simulink library "lib_vehicle"  (Simulink 4.1.1)
undefined symbols (not defined in the file or in its folder): cyc_mph, lib_help, NOTES, veh_air_density, veh_CD, veh_FA, veh_front_wt_frac, veh_gravity, veh_mass, veh_roadwheel_radius, veh_rr_a, veh_rr_alpha, veh_rr_b, veh_rr_beta, veh_rr_c, wh_1st_rrc, wh_2nd_rrc, wh_pressure, wh_radius
libraries: lib_vehicle x23
settings Model: LastModifiedBy=ssprik
settings Model: ModifiedComment=|
  | ssprik -- Fri Sep 05 12:04:31 2003 -- Version 1.64
  | added climbing grade calculation in .../vehicle speed (m/s)/ j2452/c
settings Model: ModifiedHistory=|
  | ssprik -- Fri Sep 05 12:04:31 2003 -- Version 1.64
  | added climbing grade calculation in .../vehicle speed (m/s)/ j2452/c
  | 
  | abrooker -- Fri Feb 07 11:31:15 2003 -- Version 1.63
  | 
  | 
  | abrooker -- Fri Feb 07 11:30:31 2003 -- Version 1.62
  | 
  | 
  | abrooker -- Fri Feb 07 07:46:30 2003 -- Version 1.61
  | 
  | 
  | abrooker -- Thu Feb 06 15:38:07 2003 -- Version 1.60
  | 
  | 
  | abrooker -- Thu Feb 06 14:26:47 2003 -- Version 1.59
  | changed from outputting force to power
  | 
  | abrooker -- Thu Feb 06 13:48:22 2003 -- Version 1.58
  | 
  | 
  | abrooker -- Thu Feb 06 13:42:04 2003 -- Version 1.57
  | 
  | 
  | abrooker -- Wed Feb 05 11:42:46 2003 -- Version 1.56
  | 
  | 
  | abrooker -- Wed Feb 05 11:29:37 2003 -- Version 1.55
  | 
  | 
  | abrooker -- Wed Feb 05 11:27:23 2003 -- Version 1.54
  | 
  | 
  | abrooker -- Wed Feb 05 11:19:28 2003 -- Version 1.53
  | Changed Fr_out to Fr in new rolling resistance block
  | 
  | abrooker -- Wed Feb 05 10:01:32 2003 -- Version 1.52
  | added outputs for Altia
  | 
  | mokeefe -- Thu Apr 18 08:39:48 2002 -- Version 1.51
  | saving the model:
  | o "without the model browser open"
  | o with only top-level screen visible
  | o with "fit to view" enabled
  | o with "status bar" off and "toolbar" off
  | o with "prompt to update model history with each save" on

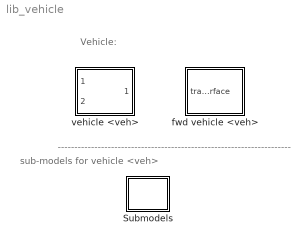
== system lib_vehicle ==
  note: Vehicle:
  note: ----------------------------------------------------------------------
  note: sub-models
      | for vehicle
      | <veh>
  Submodels : Subsystem
      settings: RTWFcnNameOpts=Auto  RTWFileNameOpts=Auto
  fwd vehicle <veh> : Subsystem
      settings: RTWFcnNameOpts=Auto  RTWFileNameOpts=Auto
      mask Display: image(imread('bdi_veh.jpg'))
  vehicle <veh> : Subsystem
      settings: RTWFcnNameOpts=Auto  RTWFileNameOpts=Auto
      mask Display: image(imread('bdi_veh.jpg'))

== system lib_vehicle/Submodels ==
  current veh mass : Subsystem
      settings: RTWFcnNameOpts=Auto  RTWFileNameOpts=Auto
  force req'd to overcome rolling resistance (N) : Subsystem
      settings: RTWFcnNameOpts=Auto  RTWFileNameOpts=Auto
  force req'd to overcome rolling resistance (N) j2452 : Subsystem
      settings: RTWFcnNameOpts=Auto  RTWFileNameOpts=Auto
  rolling resistance force : Subsystem  BlockChoice=force req'd to overcome rolling resistance (N)
      settings: TemplateBlock=self  MemberBlocks=force req'd to overcome rolling resistance (N),force req'd to overcome rolling resistance (N) j2452  RTWFcnNameOpts=Auto  RTWFileNameOpts=Auto
  vehicle speed : Subsystem  BlockChoice=vehicle speed (m/s)
      settings: TemplateBlock=self  MemberBlocks=vehicle speed (m/s),vehicle speed (m/s) j2452  RTWFcnNameOpts=Auto  RTWFileNameOpts=Auto
  vehicle speed (m/s) : Subsystem
      settings: RTWFcnNameOpts=Auto  RTWFileNameOpts=Auto
  vehicle speed (m/s) j2452 : Subsystem  AncestorBlock=|
      | lib_vehicle/Submodels/vehicle speed
      |  (m//s) j2452
      settings: RTWFcnNameOpts=Auto  RTWFileNameOpts=Auto

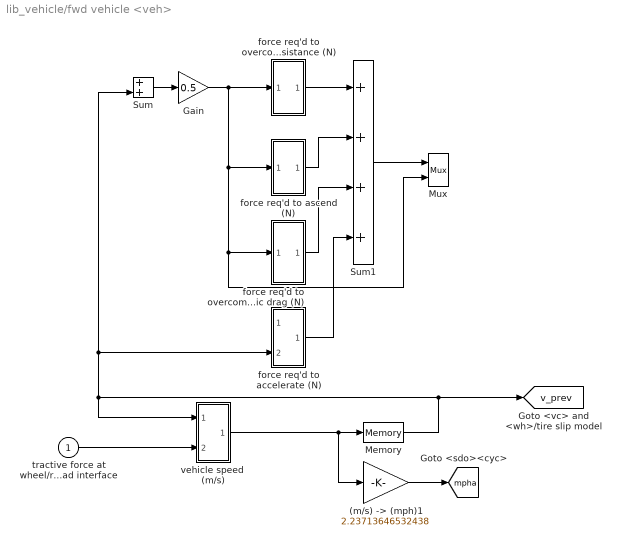
== system lib_vehicle/fwd vehicle <veh> ==
  tractive force at wheel/road interface : Inport  Port=1  LatchInput=off
  "(m/s) -> (mph)1" : Gain  Gain=2.23713646532438  Multiplication=Element-wise(K.*u)  SaturateOnIntegerOverflow=on
  Gain : Gain  Gain=0.5  Multiplication=Element-wise(K.*u)  SaturateOnIntegerOverflow=on
  Memory : Memory  X0=cyc_mph(1,2)*.447  InheritSampleTime=off
      settings: RTWStateStorageClass=Auto
  Mux : Mux  Inputs=2
      settings: DisplayOption=none
  Sum : Sum  Inputs=++  SaturateOnIntegerOverflow=on
  Sum1 : Sum  Inputs=++++  SaturateOnIntegerOverflow=on
  force req'd to accelerate (N) : Subsystem
      settings: RTWFcnNameOpts=Auto  RTWFileNameOpts=Auto
  force req'd to ascend (N) : Subsystem
      settings: RTWFcnNameOpts=Auto  RTWFileNameOpts=Auto
  force req'd to overcome aerodynamic drag (N) : Subsystem
      settings: RTWFcnNameOpts=Auto  RTWFileNameOpts=Auto
  force req'd to overcome rolling resistance (N) : Subsystem
      settings: RTWFcnNameOpts=Auto  RTWFileNameOpts=Auto
  vehicle speed  (m/s) : Subsystem
      settings: RTWFcnNameOpts=Auto  RTWFileNameOpts=Auto
  tag scope: mpha=global, v_prev=global
  wires:
  vehicle speed  (m/s)/1(vehicle speed achieved at end of time step (m/s)) -> Memory/1, "(m/s) -> (mph)1"/1
  Gain/1 -> force req'd to overcome rolling resistance (N)/1(average vehicle speed over time step (m/s)), force req'd to overcome aerodynamic drag (N)/1(average vehicle speed over time step (m/s)), Mux/2, force req'd to ascend (N)/1(average vehicle speed over time step (m/s))
  Sum/1 -> Gain/1
  force req'd to overcome aerodynamic drag (N)/1(D aero(N)) -> Sum1/3
  force req'd to accelerate (N)/1((N)) -> Sum1/4
  Memory/1 -> force req'd to accelerate (N)/2(v prev), Sum/2, vehicle speed  (m/s)/1(vehicle speed at beginning of time step (m/s)), [v_prev]
  "(m/s) -> (mph)1"/1 -> [mpha]
  force req'd to ascend (N)/1((N)) -> Sum1/2
  force req'd to overcome rolling resistance (N)/1((N)) -> Sum1/1
  tractive force at wheel/road interface/1 -> vehicle speed  (m/s)/2(available tractive force (N))
  Sum1/1 -> Mux/1

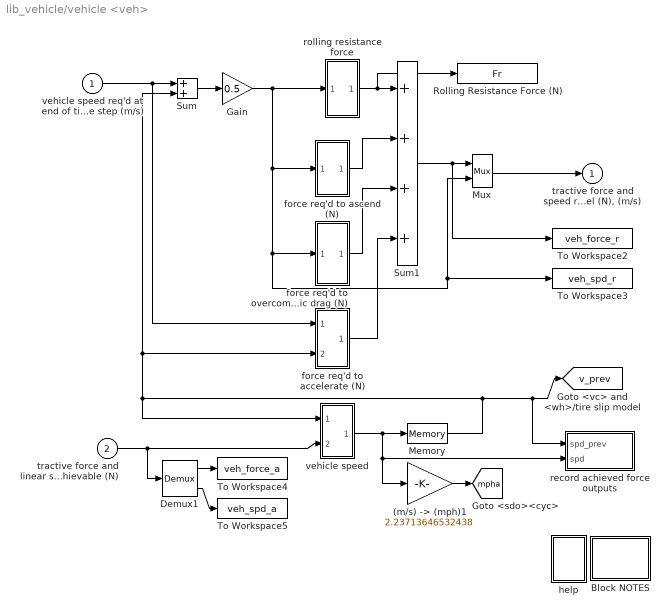
== system lib_vehicle/vehicle <veh> ==
  vehicle speed req'd at end of time step (m/s) : Inport  Port=1  LatchInput=off
  tractive force and linear speed achievable (N) : Inport  Port=2  LatchInput=off
  "(m/s) -> (mph)1" : Gain  Gain=2.23713646532438  Multiplication=Element-wise(K.*u)  SaturateOnIntegerOverflow=on
  Block NOTES : Subsystem
      settings: RTWFcnNameOpts=Auto  RTWFileNameOpts=Auto
      mask Display: disp('Block\nNOTES')
  Demux1 : Demux  Outputs=2  BusSelectionMode=off
  Gain : Gain  Gain=0.5  Multiplication=Element-wise(K.*u)  SaturateOnIntegerOverflow=on
  Memory : Memory  X0=cyc_mph(1,2)*.447  InheritSampleTime=off
      settings: RTWStateStorageClass=Auto
  Mux : Mux  Inputs=2
      settings: DisplayOption=none
  Rolling Resistance Force (N) : ToWorkspace  VariableName=Fr  SampleTime=-1  SaveFormat=Array
  Sum : Sum  Inputs=++  SaturateOnIntegerOverflow=on
  Sum1 : Sum  Inputs=++++  SaturateOnIntegerOverflow=on
  To Workspace2 : ToWorkspace  VariableName=veh_force_r  SampleTime=-1  SaveFormat=Array
  To Workspace3 : ToWorkspace  VariableName=veh_spd_r  SampleTime=-1  SaveFormat=Array
  To Workspace4 : ToWorkspace  VariableName=veh_force_a  SampleTime=-1  SaveFormat=Array
  To Workspace5 : ToWorkspace  VariableName=veh_spd_a  SampleTime=-1  SaveFormat=Array
  force req'd to accelerate (N) : Subsystem
      settings: RTWFcnNameOpts=Auto  RTWFileNameOpts=Auto
  force req'd to ascend (N) : Subsystem
      settings: RTWFcnNameOpts=Auto  RTWFileNameOpts=Auto
  force req'd to overcome aerodynamic drag (N) : Subsystem
      settings: RTWFcnNameOpts=Auto  RTWFileNameOpts=Auto
  help : Subsystem
      settings: OpenFcn=web(['file:\\\' which('vehicle.htm')]);  RTWFcnNameOpts=Auto  RTWFileNameOpts=Auto
      mask Display: image(imread('doc_man.jpg'))
  record achieved force outputs : Subsystem
      settings: RTWFcnNameOpts=Auto  RTWFileNameOpts=Auto
  rolling resistance force : Subsystem  BlockChoice=force req'd to overcome rolling resistance (N)
      settings: AttributesFormatString=%<BlockChoice>  TemplateBlock=lib_vehicle/Submodels/rolling resistance force  MemberBlocks=force req'd to overcome rolling resistance (N),force req'd to overcome rolling resistance (N) j2452  RTWFcnNameOpts=Auto  RTWFileNameOpts=Auto
  vehicle speed : Subsystem  BlockChoice=vehicle speed (m/s)
      settings: AttributesFormatString=%<BlockChoice>  TemplateBlock=lib_vehicle/Submodels/vehicle speed  MemberBlocks=vehicle speed (m/s),vehicle speed (m/s) j2452  RTWFcnNameOpts=Auto  RTWFileNameOpts=Auto
  "tractive force and speed required of tire and wheel (N), (m/s)" : Outport  Port=1  InitialOutput=0
  tag scope: mpha=global, v_prev=global
  wires:
  rolling resistance force/1(Fr (N)) -> Sum1/1, Rolling Resistance Force (N)/1
  force req'd to ascend (N)/1((N)) -> Sum1/2
  "(m/s) -> (mph)1"/1 -> [mpha]
  Memory/1 -> Sum/2, force req'd to accelerate (N)/2(v prev), vehicle speed/1(vehicle speed at beginning of time step (m/s)), [v_prev], record achieved force outputs/1(spd_prev)
  force req'd to accelerate (N)/1((N)) -> Sum1/4
  force req'd to overcome aerodynamic drag (N)/1(D aero(N)) -> Sum1/3
  Demux1/2 -> To Workspace5/1
  Demux1/1 -> To Workspace4/1
  Sum1/1 -> To Workspace2/1, Mux/1
  Mux/1 -> "tractive force and speed required of tire and wheel (N), (m/s)"/1
  vehicle speed req'd at end of time step (m/s)/1 -> Sum/1, force req'd to accelerate (N)/1(v(m/s))
  Sum/1 -> Gain/1
  Gain/1 -> force req'd to ascend (N)/1(average vehicle speed over time step (m/s)), To Workspace3/1, Mux/2, force req'd to overcome aerodynamic drag (N)/1(average vehicle speed over time step (m/s)), rolling resistance force/1(average vehicle speed over time step (m/s))
  tractive force and linear speed achievable (N)/1 -> Demux1/1, vehicle speed/2("available tractive force and linear speed (N), (m/s)")
  vehicle speed/1(vehicle speed achievable at end of time step (m/s)) -> Memory/1, "(m/s) -> (mph)1"/1, record achieved force outputs/2(spd)

== system lib_vehicle/Submodels/current veh mass ==
  Constant3 : Constant  Value=veh_mass
  Sum1 : Sum  Inputs=|++  SaturateOnIntegerOverflow=on
  Out1 : Outport  Port=1
  wires:
  Sum1/1 -> Out1/1
  [veh_cargo_mass] -> Sum1/2
  Constant3/1 -> Sum1/1

== system lib_vehicle/Submodels/force req'd to overcome rolling resistance (N) ==
  average vehicle speed over time step (m/s) : Inport  Port=1  LatchInput=off
  Constant : Constant  Value=wh_1st_rrc
  Constant1 : Constant  Orientation=up  Value=0
  Constant2 : Constant  Orientation=left  Value=veh_gravity
  Gain1 : Gain  Gain=wh_2nd_rrc  Multiplication=Element-wise(K.*u)  SaturateOnIntegerOverflow=on
  Product : Product  Inputs=4  Multiplication=Element-wise(.*)  SaturateOnIntegerOverflow=on
  Sum : Sum  Inputs=++  SaturateOnIntegerOverflow=on
  Switch : Switch  Threshold=eps
  Trig Fn2 : Trigonometry  Operator=atan  OutputSignalType=auto
  Trig Fn3 : Trigonometry  Operator=cos  OutputSignalType=auto
  current veh mass : lib_vehicle/Submodels/current veh mass
      settings: RTWFcnNameOpts=Auto  RTWFileNameOpts=Auto
  Fr (N) : Outport  Port=1  InitialOutput=0
  wires:
  Trig Fn2/1 -> Trig Fn3/1
  [grade] -> Trig Fn2/1
  current veh mass/1 -> Product/4
  Trig Fn3/1 -> Product/3
  Product/1 -> Switch/1
  Constant2/1 -> Product/1
  Sum/1 -> Product/2
  Constant1/1 -> Switch/3
  average vehicle speed over time step (m/s)/1 -> Switch/2, Gain1/1
  Switch/1 -> Fr (N)/1
  Gain1/1 -> Sum/2
  Constant/1 -> Sum/1

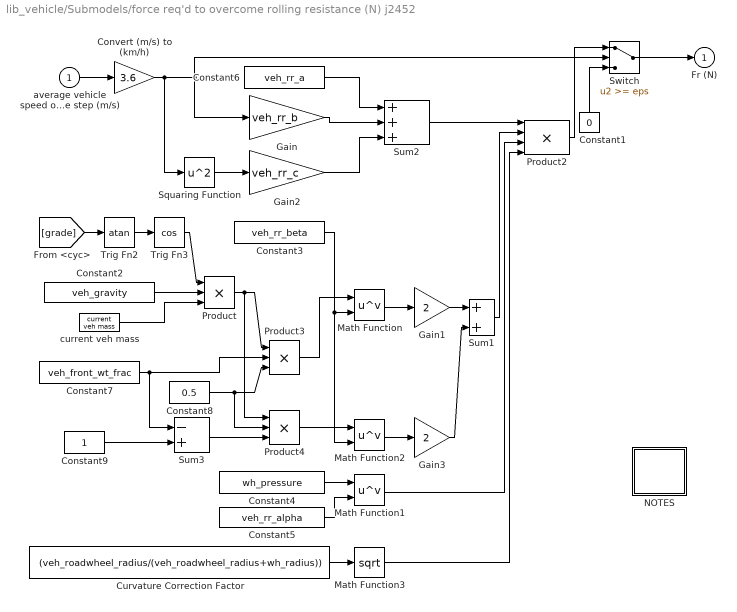
== system lib_vehicle/Submodels/force req'd to overcome rolling resistance (N) j2452 ==
  average vehicle speed over time step (m/s) : Inport  Port=1  LatchInput=off
  Constant1 : Constant  Orientation=up  Value=0
  Constant2 : Constant  Value=veh_gravity
  Constant3 : Constant  Value=veh_rr_beta
  Constant4 : Constant  Value=wh_pressure
  Constant5 : Constant  Value=veh_rr_alpha
  Constant6 : Constant  Value=veh_rr_a
  Constant7 : Constant  Value=veh_front_wt_frac
  Constant8 : Constant  Value=0.5
  Constant9 : Constant  Value=1
  Convert (m/s) to (km/h) : Gain  Description=Conversion of m/s to km/h  Gain=3.6  Multiplication=Element-wise(K.*u)  SaturateOnIntegerOverflow=on
  Curvature Correction Factor : Constant  Value=(veh_roadwheel_radius/(veh_roadwheel_radius+wh_radius))
  Gain : Gain  Gain=veh_rr_b  Multiplication=Element-wise(K.*u)  SaturateOnIntegerOverflow=on
  Gain1 : Gain  Gain=2  Multiplication=Element-wise(K.*u)  SaturateOnIntegerOverflow=on
  Gain2 : Gain  Gain=veh_rr_c  Multiplication=Element-wise(K.*u)  SaturateOnIntegerOverflow=on
  Gain3 : Gain  Gain=2  Multiplication=Element-wise(K.*u)  SaturateOnIntegerOverflow=on
  Math Function : Math  Operator=pow  OutputSignalType=auto
  Math Function1 : Math  Operator=pow  OutputSignalType=auto
  Math Function2 : Math  Operator=pow  OutputSignalType=auto
  Math Function3 : Math  Operator=sqrt  OutputSignalType=auto
  NOTES : Subsystem  Description=Notes  Orientation=left  AncestorBlock=lib_help/NOTES
      settings: RTWFcnNameOpts=Auto  RTWFileNameOpts=Auto
      mask Display: disp('Block\nNOTES')
  Product : Product  Inputs=3  Multiplication=Element-wise(.*)  SaturateOnIntegerOverflow=on
  Product2 : Product  Inputs=4  Multiplication=Element-wise(.*)  SaturateOnIntegerOverflow=on
  Product3 : Product  Inputs=3  Multiplication=Element-wise(.*)  SaturateOnIntegerOverflow=on
  Product4 : Product  Inputs=3  Multiplication=Element-wise(.*)  SaturateOnIntegerOverflow=on
  Squaring Function : Math  Operator=square  OutputSignalType=auto
  Sum1 : Sum  Inputs=++  SaturateOnIntegerOverflow=on
  Sum2 : Sum  Inputs=+++  SaturateOnIntegerOverflow=on
  Sum3 : Sum  Inputs=-+  SaturateOnIntegerOverflow=on
  Switch : Switch  Threshold=eps
  Trig Fn2 : Trigonometry  Operator=atan  OutputSignalType=auto
  Trig Fn3 : Trigonometry  Operator=cos  OutputSignalType=auto
  current veh mass : lib_vehicle/Submodels/current veh mass
      settings: RTWFcnNameOpts=Auto  RTWFileNameOpts=Auto
  Fr (N) : Outport  Port=1  InitialOutput=0
  wires:
  Curvature Correction Factor/1 -> Math Function3/1
  Math Function3/1 -> Product2/4
  Constant3/1 -> Math Function2/2, Math Function/2
  Convert (m/s) to (km/h)/1 -> Switch/2, Gain/1, Squaring Function/1
  average vehicle speed over time step (m/s)/1 -> Convert (m/s) to (km/h)/1
  Constant5/1 -> Math Function1/2
  Sum2/1 -> Product2/1
  Sum1/1 -> Product2/2
  Math Function1/1 -> Product2/3
  Gain3/1 -> Sum1/2
  Math Function2/1 -> Gain3/1
  Product4/1 -> Math Function2/1
  Sum3/1 -> Product4/3
  Constant9/1 -> Sum3/2
  Gain1/1 -> Sum1/1
  Product3/1 -> Math Function/1
  Constant8/1 -> Product4/2, Product3/3
  Constant7/1 -> Sum3/1, Product3/2
  Product/1 -> Product4/1, Product3/1
  Switch/1 -> Fr (N)/1
  Product2/1 -> Switch/1
  Gain2/1 -> Sum2/3
  Gain/1 -> Sum2/2
  Constant6/1 -> Sum2/1
  Squaring Function/1 -> Gain2/1
  Math Function/1 -> Gain1/1
  Constant4/1 -> Math Function1/1
  current veh mass/1 -> Product/3
  Constant2/1 -> Product/2
  Trig Fn3/1 -> Product/1
  [grade] -> Trig Fn2/1
  Constant1/1 -> Switch/3
  Trig Fn2/1 -> Trig Fn3/1

== system lib_vehicle/Submodels/rolling resistance force ==
  average vehicle speed over time step (m/s) : Inport  Port=1  LatchInput=off
  force req'd to overcome rolling resistance (N) : lib_vehicle/Submodels/force req'd to overcome rolling resistance (N)
      settings: RTWFcnNameOpts=Auto  RTWFileNameOpts=Auto
  Fr (N) : Outport  Port=1
  wires:
  average vehicle speed over time step (m/s)/1 -> force req'd to overcome rolling resistance (N)/1
  force req'd to overcome rolling resistance (N)/1 -> Fr (N)/1

== system lib_vehicle/Submodels/vehicle speed ==
  vehicle speed at beginning of time step (m/s) : Inport  Port=1  LatchInput=off
  "available tractive force and linear speed (N), (m/s)" : Inport  Port=2  LatchInput=off
  vehicle speed (m/s) : lib_vehicle/Submodels/vehicle speed (m//s)
      settings: RTWFcnNameOpts=Auto  RTWFileNameOpts=Auto
  vehicle speed achievable at end of time step (m/s) : Outport  Port=1
  wires:
  vehicle speed at beginning of time step (m/s)/1 -> vehicle speed (m/s)/1
  "available tractive force and linear speed (N), (m/s)"/1 -> vehicle speed (m/s)/2
  vehicle speed (m/s)/1 -> vehicle speed achievable at end of time step (m/s)/1

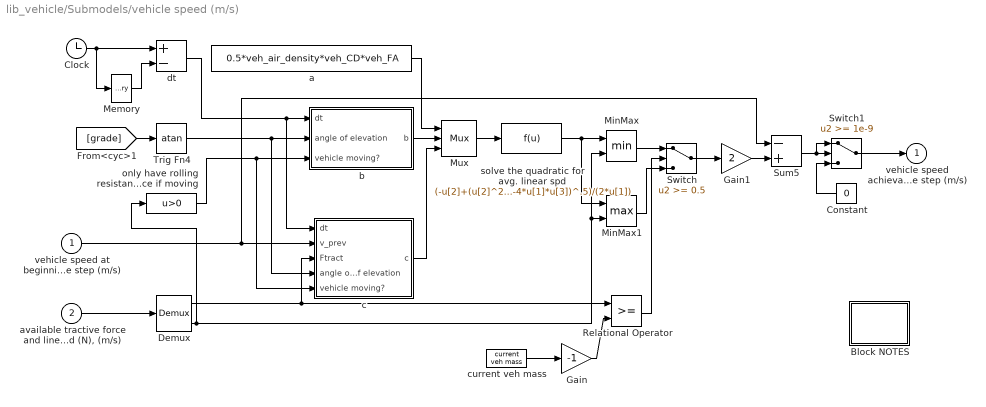
== system lib_vehicle/Submodels/vehicle speed (m/s) ==
  vehicle speed at beginning of time step (m/s) : Inport  Port=1  LatchInput=off
  "available tractive force and linear speed (N), (m/s)" : Inport  Port=2  LatchInput=off
  Block NOTES : Subsystem
      settings: RTWFcnNameOpts=Auto  RTWFileNameOpts=Auto
      mask Display: disp('Block\nNOTES')
  Clock : Clock
      settings: DisplayTime=off  Decimation=10
  Constant : Constant  Orientation=left  Value=0
  Demux : Demux  Outputs=2  BusSelectionMode=off
  Gain : Gain  Gain=-1  Multiplication=Element-wise(K.*u)  SaturateOnIntegerOverflow=on
  Gain1 : Gain  Gain=2  Multiplication=Element-wise(K.*u)  SaturateOnIntegerOverflow=on
  Memory : Memory  X0=-.1  InheritSampleTime=off
      settings: RTWStateStorageClass=Auto
  MinMax : MinMax  Function=min  Inputs=2
  MinMax1 : MinMax  Function=max  Inputs=2
  Mux : Mux  Inputs=3
      settings: DisplayOption=none
  Relational Operator : RelationalOperator  Operator=>=
  Sum5 : Sum  Inputs=-+  SaturateOnIntegerOverflow=on
  Switch : Switch  Threshold=0.5
  Switch1 : Switch  Threshold=1e-9
  Trig Fn4 : Trigonometry  Operator=atan  OutputSignalType=auto
  a : Constant  Value=0.5*veh_air_density*veh_CD*veh_FA
  b : Subsystem
      settings: RTWFcnNameOpts=Auto  RTWFileNameOpts=Auto
  c : Subsystem
      settings: RTWFcnNameOpts=Auto  RTWFileNameOpts=Auto
  current veh mass : lib_vehicle/Submodels/current veh mass
      settings: RTWFcnNameOpts=Auto  RTWFileNameOpts=Auto
  dt : Sum  Inputs=+-  SaturateOnIntegerOverflow=on
  only have rolling resistance if moving : Fcn  Expr=u>0
  solve the quadratic for avg. linear spd : Fcn  Expr=(-u[2]+(u[2]^2-4*u[1]*u[3])^.5)/(2*u[1])
  vehicle speed achievable at end of time step (m/s) : Outport  Port=1  InitialOutput=0
  wires:
  Relational Operator/1 -> Switch/2
  current veh mass/1 -> Gain/1
  Gain/1 -> Relational Operator/2
  Switch/1 -> Gain1/1
  solve the quadratic for avg. linear spd/1 -> MinMax/1, MinMax1/1
  Gain1/1 -> Sum5/2
  MinMax1/1 -> Switch/3
  MinMax/1 -> Switch/1
  a/1 -> Mux/1
  Mux/1 -> solve the quadratic for avg. linear spd/1
  Switch1/1 -> vehicle speed achievable at end of time step (m/s)/1
  b/1(b) -> Mux/2
  Clock/1 -> dt/1, Memory/1
  Memory/1 -> dt/2
  [grade] -> Trig Fn4/1
  dt/1 -> b/1(dt), c/1(dt)
  Trig Fn4/1 -> b/2(angle of elevation), c/4(angle of elevation)
  only have rolling resistance if moving/1 -> b/3(vehicle moving?), c/5(vehicle moving?)
  Sum5/1 -> Switch1/1, Switch1/2
  Constant/1 -> Switch1/3
  "available tractive force and linear speed (N), (m/s)"/1 -> Demux/1
  c/1(c) -> Mux/3
  Demux/2 -> only have rolling resistance if moving/1, MinMax/2, MinMax1/2
  Demux/1 -> Relational Operator/1, c/3(Ftract)
  vehicle speed at beginning of time step (m/s)/1 -> c/2(v_prev), Sum5/1

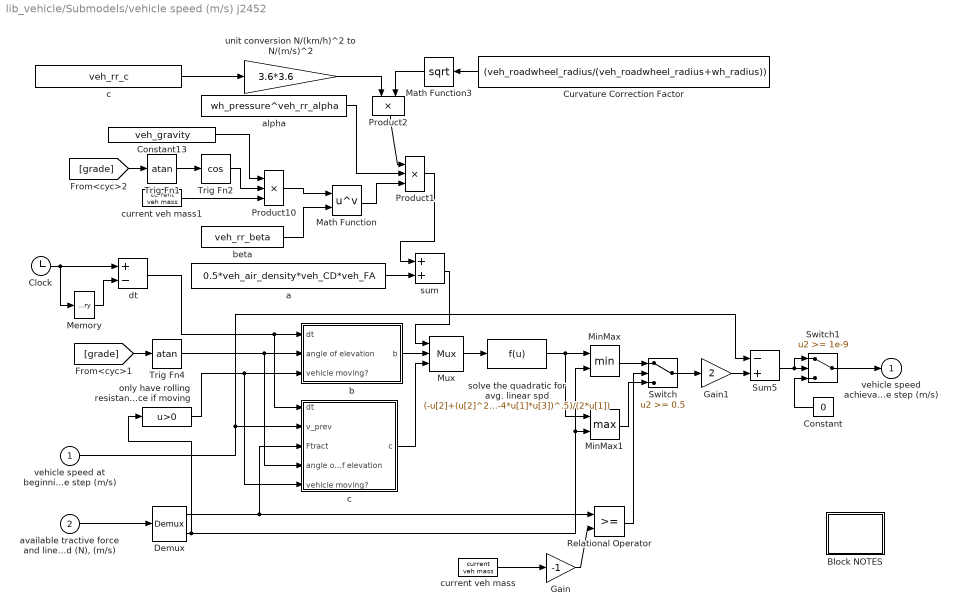
== system lib_vehicle/Submodels/vehicle speed (m/s) j2452 ==
  vehicle speed at beginning of time step (m/s) : Inport  Port=1  LatchInput=off
  "available tractive force and linear speed (N), (m/s)" : Inport  Port=2  LatchInput=off
  Block NOTES : Subsystem
      settings: RTWFcnNameOpts=Auto  RTWFileNameOpts=Auto
      mask Display: disp('Block\nNOTES')
  Clock : Clock
      settings: DisplayTime=off  Decimation=10
  Constant : Constant  Orientation=left  Value=0
  Constant13 : Constant  Value=veh_gravity
  Curvature Correction Factor : Constant  Orientation=left  Value=(veh_roadwheel_radius/(veh_roadwheel_radius+wh_radius))  VectorParams1D=off
  Demux : Demux  Outputs=2  BusSelectionMode=off
  Gain : Gain  Gain=-1  Multiplication=Element-wise(K.*u)  SaturateOnIntegerOverflow=on
  Gain1 : Gain  Gain=2  Multiplication=Element-wise(K.*u)  SaturateOnIntegerOverflow=on
  Math Function : Math  Operator=pow  OutputSignalType=auto
  Math Function3 : Math  Orientation=left  Operator=sqrt  OutputSignalType=auto
  Memory : Memory  X0=-.1  InheritSampleTime=off
      settings: RTWStateStorageClass=Auto
  MinMax : MinMax  Function=min  Inputs=2
  MinMax1 : MinMax  Function=max  Inputs=2
  Mux : Mux  Inputs=3
      settings: DisplayOption=none
  Product1 : Product  Inputs=3  Multiplication=Element-wise(.*)  SaturateOnIntegerOverflow=on
  Product10 : Product  Inputs=3  Multiplication=Element-wise(.*)  SaturateOnIntegerOverflow=on
  Product2 : Product  Orientation=down  Inputs=2  Multiplication=Element-wise(.*)  SaturateOnIntegerOverflow=on
  Relational Operator : RelationalOperator  Operator=>=
  Sum5 : Sum  Inputs=-+  SaturateOnIntegerOverflow=on
  Switch : Switch  Threshold=0.5
  Switch1 : Switch  Threshold=1e-9
  Trig Fn1 : Trigonometry  Operator=atan  OutputSignalType=auto
  Trig Fn2 : Trigonometry  Operator=cos  OutputSignalType=auto
  Trig Fn4 : Trigonometry  Operator=atan  OutputSignalType=auto
  a : Constant  Value=0.5*veh_air_density*veh_CD*veh_FA
  alpha : Constant  Value=wh_pressure^veh_rr_alpha
  b : Subsystem
      settings: RTWFcnNameOpts=Auto  RTWFileNameOpts=Auto
  beta : Constant  Value=veh_rr_beta
  c : Subsystem
      settings: RTWFcnNameOpts=Auto  RTWFileNameOpts=Auto
  "c " : Constant  Value=veh_rr_c
  current veh mass : lib_vehicle/Submodels/current veh mass
      settings: RTWFcnNameOpts=Auto  RTWFileNameOpts=Auto
  current veh mass1 : lib_vehicle/Submodels/current veh mass
      settings: RTWFcnNameOpts=Auto  RTWFileNameOpts=Auto
  dt : Sum  Inputs=+-  SaturateOnIntegerOverflow=on
  only have rolling resistance if moving : Fcn  Expr=u>0
  solve the quadratic for avg. linear spd : Fcn  Expr=(-u[2]+(u[2]^2-4*u[1]*u[3])^.5)/(2*u[1])
  sum : Sum  Inputs=++  SaturateOnIntegerOverflow=on
  unit conversion N/(km/h)^2 to N/(m/s)^2 : Gain  Gain=3.6*3.6  Multiplication=Element-wise(K.*u)  SaturateOnIntegerOverflow=on
  vehicle speed achievable at end of time step (m/s) : Outport  Port=1  InitialOutput=0
  wires:
  Product2/1 -> Product1/1
  Math Function3/1 -> Product2/2
  unit conversion N/(km/h)^2 to N/(m/s)^2/1 -> Product2/1
  Curvature Correction Factor/1 -> Math Function3/1
  current veh mass1/1 -> Product10/3
  Trig Fn2/1 -> Product10/2
  Constant13/1 -> Product10/1
  Product1/1 -> sum/1
  Math Function/1 -> Product1/3
  alpha/1 -> Product1/2
  "c "/1 -> unit conversion N/(km/h)^2 to N/(m/s)^2/1
  sum/1 -> Mux/1
  a/1 -> sum/2
  beta/1 -> Math Function/2
  Product10/1 -> Math Function/1
  Trig Fn1/1 -> Trig Fn2/1
  [grade] -> Trig Fn1/1
  vehicle speed at beginning of time step (m/s)/1 -> c/2(v_prev), Sum5/1
  Demux/1 -> c/3(Ftract), Relational Operator/1
  Demux/2 -> MinMax1/2, MinMax/2, only have rolling resistance if moving/1
  c/1(c) -> Mux/3
  "available tractive force and linear speed (N), (m/s)"/1 -> Demux/1
  Constant/1 -> Switch1/3
  Sum5/1 -> Switch1/2, Switch1/1
  only have rolling resistance if moving/1 -> c/5(vehicle moving?), b/3(vehicle moving?)
  Trig Fn4/1 -> c/4(angle of elevation), b/2(angle of elevation)
  dt/1 -> c/1(dt), b/1(dt)
  [grade] -> Trig Fn4/1
  Memory/1 -> dt/2
  Clock/1 -> Memory/1, dt/1
  b/1(b) -> Mux/2
  Switch1/1 -> vehicle speed achievable at end of time step (m/s)/1
  Mux/1 -> solve the quadratic for avg. linear spd/1
  MinMax/1 -> Switch/1
  MinMax1/1 -> Switch/3
  Gain1/1 -> Sum5/2
  solve the quadratic for avg. linear spd/1 -> MinMax1/1, MinMax/1
  Switch/1 -> Gain1/1
  Gain/1 -> Relational Operator/2
  current veh mass/1 -> Gain/1
  Relational Operator/1 -> Switch/2

== system lib_vehicle/fwd vehicle <veh>/force req'd to accelerate (N) ==
  v(m/s) : Inport  Port=1  LatchInput=off
  v prev : Inport  Port=2  LatchInput=off
  Clock : Clock
      settings: DisplayTime=off  Decimation=10
  Constant : Constant  Value=veh_mass
  Memory : Memory  X0=-0.1  InheritSampleTime=off
      settings: RTWStateStorageClass=Auto
  Product1 : Product  Inputs=**/  Multiplication=Element-wise(.*)  SaturateOnIntegerOverflow=on
  Sum : Sum  Inputs=+-  SaturateOnIntegerOverflow=on
  Sum1 : Sum  Inputs=+-  SaturateOnIntegerOverflow=on
  (N) : Outport  Port=1  InitialOutput=0
  wires:
  Constant/1 -> Product1/1
  Clock/1 -> Sum1/1, Memory/1
  Memory/1 -> Sum1/2
  Product1/1 -> (N)/1
  v prev/1 -> Sum/2
  v(m/s)/1 -> Sum/1
  Sum1/1 -> Product1/3
  Sum/1 -> Product1/2

== system lib_vehicle/fwd vehicle <veh>/force req'd to ascend (N) ==
  average vehicle speed over time step (m/s) : Inport  Port=1  LatchInput=off
  Constant : Constant  Value=veh_mass*veh_gravity
  Constant1 : Constant  Value=0
  Product : Product  Inputs=2  Multiplication=Element-wise(.*)  SaturateOnIntegerOverflow=on
  Switch : Switch  Threshold=0
  Trigonometric Function : Trigonometry  Operator=atan  OutputSignalType=auto
  Trigonometric Function1 : Trigonometry  Operator=sin  OutputSignalType=auto
  (N) : Outport  Port=1  InitialOutput=0
  wires:
  average vehicle speed over time step (m/s)/1 -> Switch/2
  Constant1/1 -> Switch/3
  Switch/1 -> (N)/1
  Product/1 -> Switch/1
  Constant/1 -> Product/1
  [grade] -> Trigonometric Function/1
  Trigonometric Function1/1 -> Product/2
  Trigonometric Function/1 -> Trigonometric Function1/1

== system lib_vehicle/fwd vehicle <veh>/force req'd to overcome aerodynamic drag (N) ==
  average vehicle speed over time step (m/s) : Inport  Port=1  LatchInput=off
  Constant : Constant  Value=veh_air_density*veh_CD*veh_FA*0.5
  Product : Product  Inputs=3  Multiplication=Element-wise(.*)  SaturateOnIntegerOverflow=on
  D aero(N) : Outport  Port=1  InitialOutput=0
  wires:
  Product/1 -> D aero(N)/1
  Constant/1 -> Product/3
  average vehicle speed over time step (m/s)/1 -> Product/2, Product/1

== system lib_vehicle/fwd vehicle <veh>/force req'd to overcome rolling resistance (N) ==
  average vehicle speed over time step (m/s) : Inport  Port=1  LatchInput=off
  Constant : Constant  Value=wh_1st_rrc
  Constant1 : Constant  Orientation=up  Value=0
  Constant2 : Constant  Orientation=left  Value=veh_mass*veh_gravity
  Gain1 : Gain  Gain=wh_2nd_rrc  Multiplication=Element-wise(K.*u)  SaturateOnIntegerOverflow=on
  Product : Product  Inputs=3  Multiplication=Element-wise(.*)  SaturateOnIntegerOverflow=on
  Sum : Sum  Inputs=++  SaturateOnIntegerOverflow=on
  Switch : Switch  Threshold=eps
  Trig Fn2 : Trigonometry  Operator=atan  OutputSignalType=auto
  Trig Fn3 : Trigonometry  Operator=cos  OutputSignalType=auto
  (N) : Outport  Port=1  InitialOutput=0
  wires:
  Trig Fn3/1 -> Product/3
  Trig Fn2/1 -> Trig Fn3/1
  [grade] -> Trig Fn2/1
  Product/1 -> Switch/1
  Constant2/1 -> Product/1
  Sum/1 -> Product/2
  Constant1/1 -> Switch/3
  average vehicle speed over time step (m/s)/1 -> Switch/2, Gain1/1
  Switch/1 -> (N)/1
  Gain1/1 -> Sum/2
  Constant/1 -> Sum/1

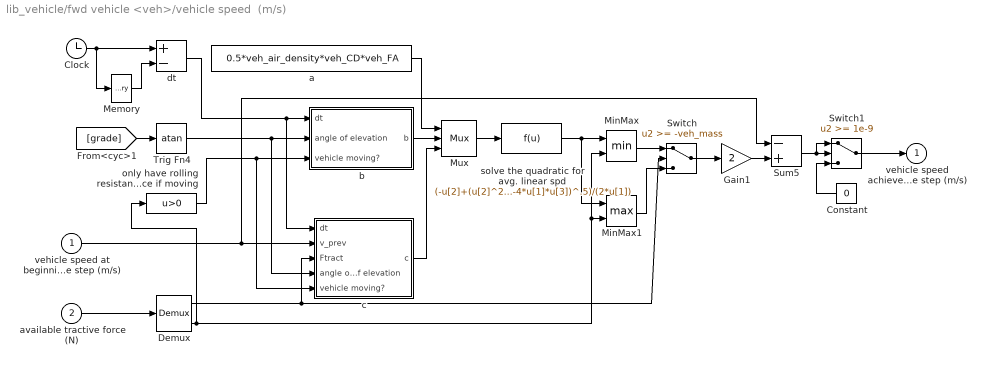
== system lib_vehicle/fwd vehicle <veh>/vehicle speed  (m/s) ==
  vehicle speed at beginning of time step (m/s) : Inport  Port=1  LatchInput=off
  available tractive force (N) : Inport  Port=2  LatchInput=off
  Clock : Clock
      settings: DisplayTime=off  Decimation=10
  Constant : Constant  Orientation=left  Value=0
  Demux : Demux  Outputs=2  BusSelectionMode=off
  Gain1 : Gain  Gain=2  Multiplication=Element-wise(K.*u)  SaturateOnIntegerOverflow=on
  Memory : Memory  X0=-.1  InheritSampleTime=off
      settings: RTWStateStorageClass=Auto
  MinMax : MinMax  Function=min  Inputs=2
  MinMax1 : MinMax  Function=max  Inputs=2
  Mux : Mux  Inputs=3
      settings: DisplayOption=none
  Sum5 : Sum  Inputs=-+  SaturateOnIntegerOverflow=on
  Switch : Switch  Threshold=-veh_mass
  Switch1 : Switch  Threshold=1e-9
  Trig Fn4 : Trigonometry  Operator=atan  OutputSignalType=auto
  a : Constant  Value=0.5*veh_air_density*veh_CD*veh_FA
  b : Subsystem
      settings: RTWFcnNameOpts=Auto  RTWFileNameOpts=Auto
  c : Subsystem
      settings: RTWFcnNameOpts=Auto  RTWFileNameOpts=Auto
  dt : Sum  Inputs=+-  SaturateOnIntegerOverflow=on
  only have rolling resistance if moving : Fcn  Expr=u>0
  solve the quadratic for avg. linear spd : Fcn  Expr=(-u[2]+(u[2]^2-4*u[1]*u[3])^.5)/(2*u[1])
  vehicle speed achieved at end of time step (m/s) : Outport  Port=1  InitialOutput=0
  wires:
  Switch/1 -> Gain1/1
  solve the quadratic for avg. linear spd/1 -> MinMax/1, MinMax1/1
  Gain1/1 -> Sum5/2
  MinMax1/1 -> Switch/3
  MinMax/1 -> Switch/1
  a/1 -> Mux/1
  Mux/1 -> solve the quadratic for avg. linear spd/1
  Switch1/1 -> vehicle speed achieved at end of time step (m/s)/1
  b/1(b) -> Mux/2
  Clock/1 -> dt/1, Memory/1
  Memory/1 -> dt/2
  [grade] -> Trig Fn4/1
  dt/1 -> b/1(dt), c/1(dt)
  Trig Fn4/1 -> b/2(angle of elevation), c/4(angle of elevation)
  only have rolling resistance if moving/1 -> b/3(vehicle moving?), c/5(vehicle moving?)
  Sum5/1 -> Switch1/1, Switch1/2
  Constant/1 -> Switch1/3
  available tractive force (N)/1 -> Demux/1
  c/1(c) -> Mux/3
  Demux/2 -> only have rolling resistance if moving/1, MinMax/2, MinMax1/2
  Demux/1 -> c/3(Ftract), Switch/2
  vehicle speed at beginning of time step (m/s)/1 -> c/2(v_prev), Sum5/1

== system lib_vehicle/vehicle <veh>/Block NOTES ==
  note: Given the tractive force available, this block uses the same equations to determine the achievable speed.
  note: If no drivetrain component ran up against its performance limit during the time step, the achieved speed
      | is taken to be the requested speed.
  note: This block uses the required vehicle speed with vehicle parameters and the previous speed
      | and classic, straightforward equations to determine the tractive force required at the tire/road interface.
  note: A slight simplification, the assumption that (speed_at_end_of_time_step)^2 is roughly equal to
      | (speed_at_end_of_time_step)*(speed_at_beginning_of_time_step), is used to avoid solving
      | a quadratic equation in the solution of v=v(Ftract).

== system lib_vehicle/vehicle <veh>/force req'd to accelerate (N) ==
  v(m/s) : Inport  Port=1  LatchInput=off
  v prev : Inport  Port=2  LatchInput=off
  Clock : Clock
      settings: DisplayTime=off  Decimation=10
  Memory : Memory  X0=-0.1  InheritSampleTime=off
      settings: RTWStateStorageClass=Auto
  Product1 : Product  Inputs=**/  Multiplication=Element-wise(.*)  SaturateOnIntegerOverflow=on
  Sum : Sum  Inputs=+-  SaturateOnIntegerOverflow=on
  Sum1 : Sum  Inputs=+-  SaturateOnIntegerOverflow=on
  current veh mass : lib_vehicle/Submodels/current veh mass
  (N) : Outport  Port=1  InitialOutput=0
  wires:
  Sum/1 -> Product1/2
  Sum1/1 -> Product1/3
  v(m/s)/1 -> Sum/1
  v prev/1 -> Sum/2
  Product1/1 -> (N)/1
  Memory/1 -> Sum1/2
  Clock/1 -> Memory/1, Sum1/1
  current veh mass/1 -> Product1/1

== system lib_vehicle/vehicle <veh>/force req'd to ascend (N) ==
  average vehicle speed over time step (m/s) : Inport  Port=1  LatchInput=off
  Constant : Constant  Value=veh_gravity
  Constant1 : Constant  Value=0
  Product : Product  Inputs=3  Multiplication=Element-wise(.*)  SaturateOnIntegerOverflow=on
  Switch : Switch  Threshold=0
  Trigonometric Function : Trigonometry  Operator=atan  OutputSignalType=auto
  Trigonometric Function1 : Trigonometry  Operator=sin  OutputSignalType=auto
  current veh mass : lib_vehicle/Submodels/current veh mass
      settings: RTWFcnNameOpts=Auto  RTWFileNameOpts=Auto
  (N) : Outport  Port=1  InitialOutput=0
  wires:
  Trigonometric Function/1 -> Trigonometric Function1/1
  Trigonometric Function1/1 -> Product/2
  [grade] -> Trigonometric Function/1
  Constant/1 -> Product/1
  Product/1 -> Switch/1
  Switch/1 -> (N)/1
  Constant1/1 -> Switch/3
  average vehicle speed over time step (m/s)/1 -> Switch/2
  current veh mass/1 -> Product/3

== system lib_vehicle/vehicle <veh>/force req'd to overcome aerodynamic drag (N) ==
  average vehicle speed over time step (m/s) : Inport  Port=1  LatchInput=off
  Constant : Constant  Value=veh_air_density*veh_CD*veh_FA*0.5
  Product : Product  Inputs=3  Multiplication=Element-wise(.*)  SaturateOnIntegerOverflow=on
  D aero(N) : Outport  Port=1  InitialOutput=0
  wires:
  average vehicle speed over time step (m/s)/1 -> Product/1, Product/2
  Constant/1 -> Product/3
  Product/1 -> D aero(N)/1

== system lib_vehicle/vehicle <veh>/help ==

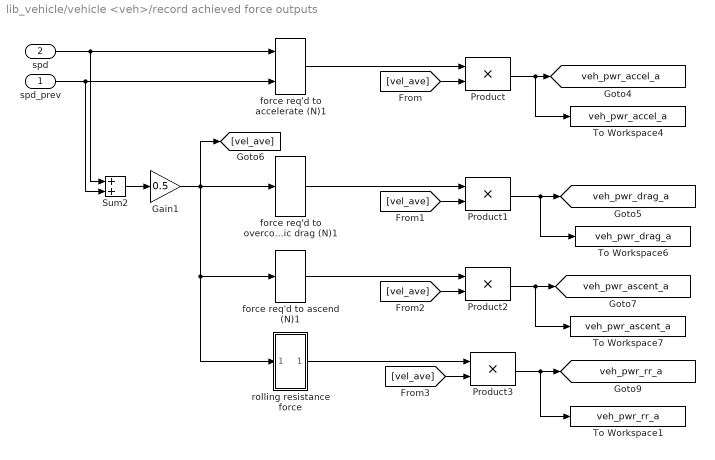
== system lib_vehicle/vehicle <veh>/record achieved force outputs ==
  spd_prev : Inport  Port=1  LatchInput=off
  spd : Inport  Port=2  LatchInput=off
  Gain1 : Gain  Gain=0.5  Multiplication=Element-wise(K.*u)  SaturateOnIntegerOverflow=on
  Product{,1..3} (4 alike) : Product  Inputs=2  Multiplication=Element-wise(.*)  SaturateOnIntegerOverflow=on
  Sum2 : Sum  Inputs=++  SaturateOnIntegerOverflow=on
  To Workspace1 : ToWorkspace  VariableName=veh_pwr_rr_a  SampleTime=-1  SaveFormat=Array
  To Workspace4 : ToWorkspace  VariableName=veh_pwr_accel_a  SampleTime=-1  SaveFormat=Array
  To Workspace6 : ToWorkspace  VariableName=veh_pwr_drag_a  SampleTime=-1  SaveFormat=Array
  To Workspace7 : ToWorkspace  VariableName=veh_pwr_ascent_a  SampleTime=-1  SaveFormat=Array
  force req'd to accelerate (N)1 : lib_vehicle/vehicle <veh>/force req'd to accelerate (N)
      settings: RTWFcnNameOpts=Auto  RTWFileNameOpts=Auto
  force req'd to ascend (N)1 : lib_vehicle/vehicle <veh>/force req'd to ascend (N)
      settings: RTWFcnNameOpts=Auto  RTWFileNameOpts=Auto
  force req'd to overcome aerodynamic drag (N)1 : lib_vehicle/vehicle <veh>/force req'd to overcome aerodynamic drag (N)
      settings: RTWFcnNameOpts=Auto  RTWFileNameOpts=Auto
  rolling resistance force : Subsystem  BlockChoice=force req'd to overcome rolling resistance (N)
      settings: AttributesFormatString=%<BlockChoice>  TemplateBlock=lib_vehicle/Submodels/rolling resistance force  MemberBlocks=force req'd to overcome rolling resistance (N),force req'd to overcome rolling resistance (N) j2452  RTWFcnNameOpts=Auto  RTWFileNameOpts=Auto
  tag scope: veh_pwr_accel_a=global, veh_pwr_ascent_a=global, veh_pwr_drag_a=global, veh_pwr_rr_a=global
  wires:
  Sum2/1 -> Gain1/1
  spd/1 -> force req'd to accelerate (N)1/1, Sum2/1
  spd_prev/1 -> force req'd to accelerate (N)1/2, Sum2/2
  force req'd to overcome aerodynamic drag (N)1/1 -> Product1/1
  force req'd to ascend (N)1/1 -> Product2/1
  rolling resistance force/1(Fr (N)) -> Product3/1
  force req'd to accelerate (N)1/1 -> Product/1
  Product/1 -> To Workspace4/1, [veh_pwr_accel_a]
  Product1/1 -> To Workspace6/1, [veh_pwr_drag_a]
  [vel_ave] -> Product/2
  [vel_ave] -> Product1/2
  [vel_ave] -> Product2/2
  Product2/1 -> To Workspace7/1, [veh_pwr_ascent_a]
  [vel_ave] -> Product3/2
  Product3/1 -> [veh_pwr_rr_a], To Workspace1/1
  Gain1/1 -> force req'd to overcome aerodynamic drag (N)1/1, force req'd to ascend (N)1/1, rolling resistance force/1(average vehicle speed over time step (m/s)), [vel_ave]

== system lib_vehicle/vehicle <veh>/rolling resistance force ==
  average vehicle speed over time step (m/s) : Inport  Port=1  LatchInput=off
  force req'd to overcome rolling resistance (N) : lib_vehicle/Submodels/force req'd to overcome rolling resistance (N)
      settings: RTWFcnNameOpts=Auto  RTWFileNameOpts=Auto
  Fr (N) : Outport  Port=1
  wires:
  average vehicle speed over time step (m/s)/1 -> force req'd to overcome rolling resistance (N)/1
  force req'd to overcome rolling resistance (N)/1 -> Fr (N)/1

== system lib_vehicle/vehicle <veh>/vehicle speed ==
  vehicle speed at beginning of time step (m/s) : Inport  Port=1  LatchInput=off
  "available tractive force and linear speed (N), (m/s)" : Inport  Port=2  LatchInput=off
  vehicle speed (m/s) : lib_vehicle/Submodels/vehicle speed (m//s)
      settings: RTWFcnNameOpts=Auto  RTWFileNameOpts=Auto
  vehicle speed achievable at end of time step (m/s) : Outport  Port=1
  wires:
  vehicle speed at beginning of time step (m/s)/1 -> vehicle speed (m/s)/1
  "available tractive force and linear speed (N), (m/s)"/1 -> vehicle speed (m/s)/2
  vehicle speed (m/s)/1 -> vehicle speed achievable at end of time step (m/s)/1

== system lib_vehicle/Submodels/force req'd to overcome rolling resistance (N) j2452/NOTES ==
  note: Rolling resistance model updated to SAE J2452 model.
      | Fr = (P^alpha)*(a + bV + cV^2)*[2((mg*veh_front_wt_frac/2)^beta) + 2((mg(1-veh_front_wt_frac)/2)^beta)]
      | Incorporates pressure, load, and velocity into rolling resistance.
      |
      | Alpha, beta, a, b, and c were for curved surface rolling resistance.
      | Curvature correction factor from SAE J2452 [Eq. 22] added to relate to flat surface rolling resistance.
      | This is an approximation for convenience, but the error is fairly small.

== system lib_vehicle/Submodels/vehicle speed (m/s)/Block NOTES ==
  note: The actual vehicle speed at the end of the time step is taken as
      | the LESSER of the speed computed from the actual force and the speed
      | computed from the actual drivetrain speed if the required acceleration
      |  is greater than -1 m/s^2.  Otherwise, the GREATER of the two values is used.
      | Thus the worse acceleration rate is allowed if the vehicle is accelerating,
      | and the worse deceleration rate is allowed if the vehicle is decelerating.
      |
      | In no case will the computed speed fall below zero.
  note: Given the tractive force available, this block uses straightforward vehicle
      | dynamics equations to determine the achievable speed.

== system lib_vehicle/Submodels/vehicle speed (m/s)/b ==
  dt : Inport  Port=1  LatchInput=off
  angle of elevation : Inport  Port=2  LatchInput=off
  vehicle moving? : Inport  Port=3  LatchInput=off
  Constant9 : Constant  Value=veh_gravity*wh_2nd_rrc
  Gain : Gain  Gain=2  Multiplication=Element-wise(K.*u)  SaturateOnIntegerOverflow=on
  Product10 : Product  Inputs=4  Multiplication=Element-wise(.*)  SaturateOnIntegerOverflow=on
  Product6 : Product  Inputs=*/  Multiplication=Element-wise(.*)  SaturateOnIntegerOverflow=on
  Sum : Sum  Inputs=++  SaturateOnIntegerOverflow=on
  Trig Fn7 : Trigonometry  Operator=cos  OutputSignalType=auto
  current veh mass : lib_vehicle/Submodels/current veh mass
      settings: RTWFcnNameOpts=Auto  RTWFileNameOpts=Auto
  current veh mass1 : lib_vehicle/Submodels/current veh mass
      settings: RTWFcnNameOpts=Auto  RTWFileNameOpts=Auto
  b : Outport  Port=1
  wires:
  current veh mass1/1 -> Product10/4
  current veh mass/1 -> Gain/1
  vehicle moving?/1 -> Product10/3
  angle of elevation/1 -> Trig Fn7/1
  dt/1 -> Product6/2
  Sum/1 -> b/1
  Product10/1 -> Sum/2
  Constant9/1 -> Product10/1
  Trig Fn7/1 -> Product10/2
  Product6/1 -> Sum/1
  Gain/1 -> Product6/1

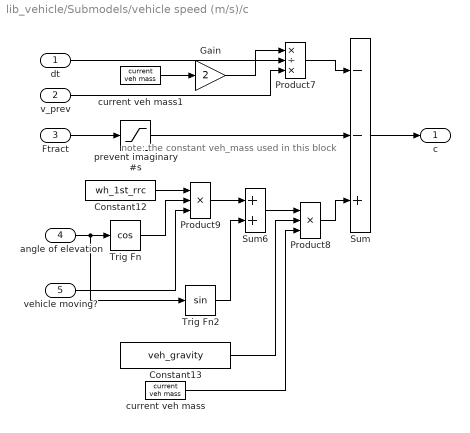
== system lib_vehicle/Submodels/vehicle speed (m/s)/c ==
  note: note: the constant
      | veh_mass used in this block
  dt : Inport  Port=1  LatchInput=off
  v_prev : Inport  Port=2  LatchInput=off
  Ftract : Inport  Port=3  LatchInput=off
  angle of elevation : Inport  Port=4  LatchInput=off
  vehicle moving? : Inport  Port=5  LatchInput=off
  Constant12 : Constant  Value=wh_1st_rrc
  Constant13 : Constant  Value=veh_gravity
  Gain : Gain  Gain=2  Multiplication=Element-wise(K.*u)  SaturateOnIntegerOverflow=on
  Product7 : Product  Inputs=*/*  Multiplication=Element-wise(.*)  SaturateOnIntegerOverflow=on
  Product8 : Product  Inputs=3  Multiplication=Element-wise(.*)  SaturateOnIntegerOverflow=on
  Product9 : Product  Inputs=3  Multiplication=Element-wise(.*)  SaturateOnIntegerOverflow=on
  Sum : Sum  Inputs=--+  SaturateOnIntegerOverflow=on
  Sum6 : Sum  Inputs=++  SaturateOnIntegerOverflow=on
  Trig Fn : Trigonometry  Operator=cos  OutputSignalType=auto
  Trig Fn2 : Trigonometry  Operator=sin  OutputSignalType=auto
  current veh mass : lib_vehicle/Submodels/current veh mass
      settings: RTWFcnNameOpts=Auto  RTWFileNameOpts=Auto
  current veh mass1 : lib_vehicle/Submodels/current veh mass
      settings: RTWFcnNameOpts=Auto  RTWFileNameOpts=Auto
  prevent imaginary #s : Saturate  UpperLimit=inf  LowerLimit=-70*veh_mass  LinearizeAsGain=on
  c : Outport  Port=1
  wires:
  current veh mass/1 -> Product8/3
  current veh mass1/1 -> Gain/1
  Gain/1 -> Product7/1
  dt/1 -> Product7/2
  Sum/1 -> c/1
  Product8/1 -> Sum/3
  Constant13/1 -> Product8/2
  Sum6/1 -> Product8/1
  vehicle moving?/1 -> Product9/3
  Trig Fn2/1 -> Sum6/2
  angle of elevation/1 -> Trig Fn2/1, Trig Fn/1
  Product9/1 -> Sum6/1
  Trig Fn/1 -> Product9/2
  Constant12/1 -> Product9/1
  Ftract/1 -> prevent imaginary #s/1
  prevent imaginary #s/1 -> Sum/2
  Product7/1 -> Sum/1
  v_prev/1 -> Product7/3

== system lib_vehicle/Submodels/vehicle speed (m/s) j2452/Block NOTES ==
  note: Rolling resistance force was brought into model to solve the quadratic.
      | Veh_rr_b and veh_rr_c were converted to the proper units.
  note: Given the tractive force available, this block uses straightforward vehicle
      | dynamics equations to determine the achievable speed.
  note: The actual vehicle speed at the end of the time step is taken as
      | the LESSER of the speed computed from the actual force and the speed
      | computed from the actual drivetrain speed if the required acceleration
      |  is greater than -1 m/s^2.  Otherwise, the GREATER of the two values is used.
      | Thus the worse acceleration rate is allowed if the vehicle is accelerating,
      | and the worse deceleration rate is allowed if the vehicle is decelerating.
      |
      | In no case will the computed speed fall below zero.

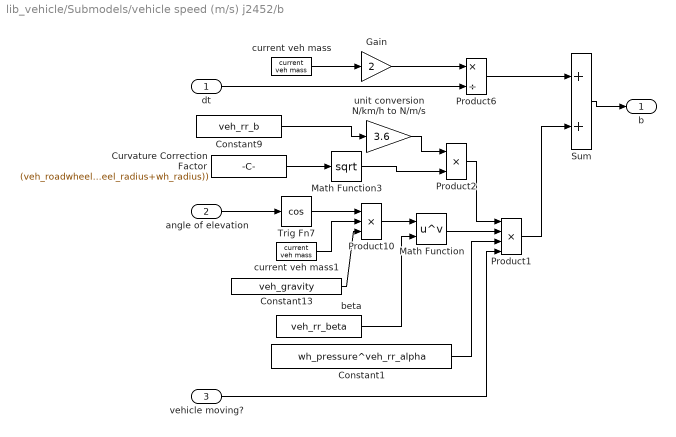
== system lib_vehicle/Submodels/vehicle speed (m/s) j2452/b ==
  dt : Inport  Port=1  LatchInput=off
  angle of elevation : Inport  Port=2  LatchInput=off
  vehicle moving? : Inport  Port=3  LatchInput=off
  Constant1 : Constant  Value=wh_pressure^veh_rr_alpha  VectorParams1D=off
  Constant13 : Constant  Value=veh_gravity
  Constant9 : Constant  Value=veh_rr_b  VectorParams1D=off
  Curvature Correction Factor : Constant  Value=(veh_roadwheel_radius/(veh_roadwheel_radius+wh_radius))  VectorParams1D=off
  Gain : Gain  Gain=2  Multiplication=Element-wise(K.*u)  SaturateOnIntegerOverflow=on
  Math Function : Math  Operator=pow  OutputSignalType=auto
  Math Function3 : Math  Operator=sqrt  OutputSignalType=auto
  Product1 : Product  Inputs=4  Multiplication=Element-wise(.*)  SaturateOnIntegerOverflow=on
  Product10 : Product  Inputs=3  Multiplication=Element-wise(.*)  SaturateOnIntegerOverflow=on
  Product2 : Product  Inputs=2  Multiplication=Element-wise(.*)  SaturateOnIntegerOverflow=on
  Product6 : Product  Inputs=*/  Multiplication=Element-wise(.*)  SaturateOnIntegerOverflow=on
  Sum : Sum  Inputs=++  SaturateOnIntegerOverflow=on
  Trig Fn7 : Trigonometry  Operator=cos  OutputSignalType=auto
  beta : Constant  Value=veh_rr_beta
  current veh mass : lib_vehicle/Submodels/current veh mass
      settings: RTWFcnNameOpts=Auto  RTWFileNameOpts=Auto
  current veh mass1 : lib_vehicle/Submodels/current veh mass
      settings: RTWFcnNameOpts=Auto  RTWFileNameOpts=Auto
  unit conversion N/km/h to N/m/s : Gain  Gain=3.6  Multiplication=Element-wise(K.*u)  SaturateOnIntegerOverflow=on
  b : Outport  Port=1
  wires:
  Product2/1 -> Product1/1
  Math Function3/1 -> Product2/2
  unit conversion N/km/h to N/m/s/1 -> Product2/1
  Curvature Correction Factor/1 -> Math Function3/1
  Constant13/1 -> Product10/3
  Product1/1 -> Sum/2
  vehicle moving?/1 -> Product1/4
  Constant1/1 -> Product1/3
  Math Function/1 -> Product1/2
  Constant9/1 -> unit conversion N/km/h to N/m/s/1
  beta/1 -> Math Function/2
  Product10/1 -> Math Function/1
  current veh mass1/1 -> Product10/2
  Trig Fn7/1 -> Product10/1
  Gain/1 -> Product6/1
  Product6/1 -> Sum/1
  Sum/1 -> b/1
  dt/1 -> Product6/2
  angle of elevation/1 -> Trig Fn7/1
  current veh mass/1 -> Gain/1

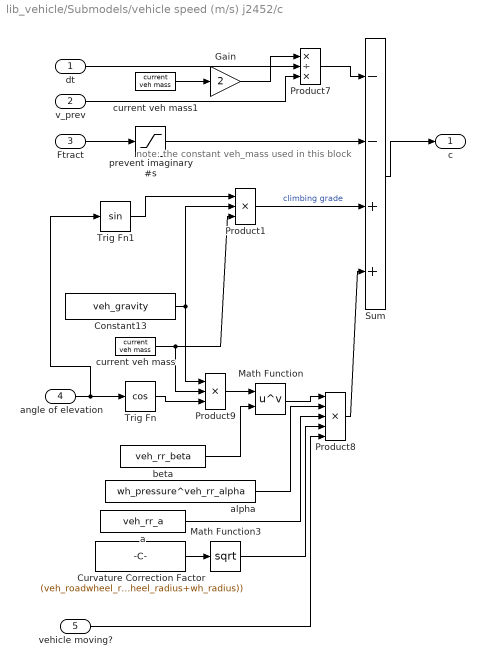
== system lib_vehicle/Submodels/vehicle speed (m/s) j2452/c ==
  note: note: the constant
      | veh_mass used in this block
  dt : Inport  Port=1  LatchInput=off
  v_prev : Inport  Port=2  LatchInput=off
  Ftract : Inport  Port=3  LatchInput=off
  angle of elevation : Inport  Port=4  LatchInput=off
  vehicle moving? : Inport  Port=5  LatchInput=off
  Constant13 : Constant  Value=veh_gravity
  Curvature Correction Factor : Constant  Value=(veh_roadwheel_radius/(veh_roadwheel_radius+wh_radius))  VectorParams1D=off
  Gain : Gain  Gain=2  Multiplication=Element-wise(K.*u)  SaturateOnIntegerOverflow=on
  Math Function : Math  Operator=pow  OutputSignalType=auto
  Math Function3 : Math  Operator=sqrt  OutputSignalType=auto
  Product1 : Product  Inputs=3  Multiplication=Element-wise(.*)  SaturateOnIntegerOverflow=on
  Product7 : Product  Inputs=*/*  Multiplication=Element-wise(.*)  SaturateOnIntegerOverflow=on
  Product8 : Product  Inputs=5  Multiplication=Element-wise(.*)  SaturateOnIntegerOverflow=on
  Product9 : Product  Inputs=3  Multiplication=Element-wise(.*)  SaturateOnIntegerOverflow=on
  Sum : Sum  Inputs=--++  SaturateOnIntegerOverflow=on
  Trig Fn : Trigonometry  Operator=cos  OutputSignalType=auto
  Trig Fn1 : Trigonometry  Operator=sin  OutputSignalType=auto
  a : Constant  Value=veh_rr_a
  alpha : Constant  Value=wh_pressure^veh_rr_alpha
  beta : Constant  Value=veh_rr_beta
  current veh mass : lib_vehicle/Submodels/current veh mass
      settings: RTWFcnNameOpts=Auto  RTWFileNameOpts=Auto
  current veh mass1 : lib_vehicle/Submodels/current veh mass
      settings: RTWFcnNameOpts=Auto  RTWFileNameOpts=Auto
  prevent imaginary #s : Saturate  UpperLimit=inf  LowerLimit=-70*veh_mass  LinearizeAsGain=on
  c : Outport  Port=1
  wires:
  vehicle moving?/1 -> Product8/5
  Math Function3/1 -> Product8/4
  Curvature Correction Factor/1 -> Math Function3/1
  a/1 -> Product8/3
  alpha/1 -> Product8/2
  Math Function/1 -> Product8/1
  beta/1 -> Math Function/2
  Product9/1 -> Math Function/1
  Trig Fn/1 -> Product9/3
  current veh mass/1 -> Product9/2, Product1/3
  Constant13/1 -> Product9/1, Product1/2
  v_prev/1 -> Product7/3
  Product7/1 -> Sum/1
  prevent imaginary #s/1 -> Sum/2
  Ftract/1 -> prevent imaginary #s/1
  angle of elevation/1 -> Trig Fn/1, Trig Fn1/1
  Sum/1 -> c/1
  dt/1 -> Product7/2
  Gain/1 -> Product7/1
  current veh mass1/1 -> Gain/1
  Product8/1 -> Sum/4
  Product1/1 -> Sum/3  "climbing grade"
  Trig Fn1/1 -> Product1/1

== system lib_vehicle/fwd vehicle <veh>/vehicle speed  (m/s)/b ==
  dt : Inport  Port=1  LatchInput=off
  angle of elevation : Inport  Port=2  LatchInput=off
  vehicle moving? : Inport  Port=3  LatchInput=off
  Constant8 : Constant  Value=2*veh_mass
  Constant9 : Constant  Value=veh_mass*veh_gravity*wh_2nd_rrc
  Product10 : Product  Inputs=3  Multiplication=Element-wise(.*)  SaturateOnIntegerOverflow=on
  Product6 : Product  Inputs=*/  Multiplication=Element-wise(.*)  SaturateOnIntegerOverflow=on
  Sum : Sum  Inputs=++  SaturateOnIntegerOverflow=on
  Trig Fn7 : Trigonometry  Operator=cos  OutputSignalType=auto
  b : Outport  Port=1
  wires:
  vehicle moving?/1 -> Product10/3
  angle of elevation/1 -> Trig Fn7/1
  dt/1 -> Product6/2
  Sum/1 -> b/1
  Product10/1 -> Sum/2
  Constant9/1 -> Product10/1
  Trig Fn7/1 -> Product10/2
  Product6/1 -> Sum/1
  Constant8/1 -> Product6/1

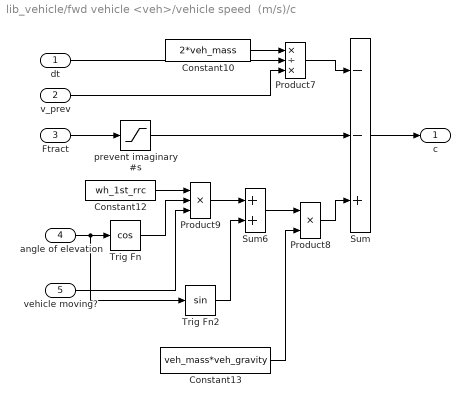
== system lib_vehicle/fwd vehicle <veh>/vehicle speed  (m/s)/c ==
  dt : Inport  Port=1  LatchInput=off
  v_prev : Inport  Port=2  LatchInput=off
  Ftract : Inport  Port=3  LatchInput=off
  angle of elevation : Inport  Port=4  LatchInput=off
  vehicle moving? : Inport  Port=5  LatchInput=off
  Constant10 : Constant  Value=2*veh_mass
  Constant12 : Constant  Value=wh_1st_rrc
  Constant13 : Constant  Value=veh_mass*veh_gravity
  Product7 : Product  Inputs=*/*  Multiplication=Element-wise(.*)  SaturateOnIntegerOverflow=on
  Product8 : Product  Inputs=2  Multiplication=Element-wise(.*)  SaturateOnIntegerOverflow=on
  Product9 : Product  Inputs=3  Multiplication=Element-wise(.*)  SaturateOnIntegerOverflow=on
  Sum : Sum  Inputs=--+  SaturateOnIntegerOverflow=on
  Sum6 : Sum  Inputs=++  SaturateOnIntegerOverflow=on
  Trig Fn : Trigonometry  Operator=cos  OutputSignalType=auto
  Trig Fn2 : Trigonometry  Operator=sin  OutputSignalType=auto
  prevent imaginary #s : Saturate  UpperLimit=inf  LowerLimit=-70*veh_mass  LinearizeAsGain=on
  c : Outport  Port=1
  wires:
  Sum/1 -> c/1
  Product8/1 -> Sum/3
  Constant13/1 -> Product8/2
  Sum6/1 -> Product8/1
  vehicle moving?/1 -> Product9/3
  Trig Fn2/1 -> Sum6/2
  angle of elevation/1 -> Trig Fn2/1, Trig Fn/1
  Product9/1 -> Sum6/1
  Trig Fn/1 -> Product9/2
  Constant12/1 -> Product9/1
  Ftract/1 -> prevent imaginary #s/1
  prevent imaginary #s/1 -> Sum/2
  Product7/1 -> Sum/1
  v_prev/1 -> Product7/3
  dt/1 -> Product7/2
  Constant10/1 -> Product7/1

== system lib_vehicle/vehicle <veh>/record achieved force outputs/rolling resistance force ==
  average vehicle speed over time step (m/s) : Inport  Port=1  LatchInput=off
  force req'd to overcome rolling resistance (N) : lib_vehicle/Submodels/force req'd to overcome rolling resistance (N)
      settings: RTWFcnNameOpts=Auto  RTWFileNameOpts=Auto
  Fr (N) : Outport  Port=1
  wires:
  average vehicle speed over time step (m/s)/1 -> force req'd to overcome rolling resistance (N)/1
  force req'd to overcome rolling resistance (N)/1 -> Fr (N)/1
